simulink model "CrCtl_Governor"  (R2016b)
settings: configuration reference "CodeGenConfigSet" (kept outside this file)
values from neighbouring files (symbols this model uses):
  ACC_ZERO = fi(0,Acc_m_s2)    [init_CrCtl_Governor.m]
  CrCtl_facAcc2TrqCor_C = Calibration.Parameter    [init_CrCtl_Governor.m]
  CrCtl_facDecl2TrqCor_C = Calibration.Parameter    [init_CrCtl_Governor.m]
  CrCtl_facPT11_C = Calibration.Parameter    [init_CrCtl_Governor.m]
  CrCtl_facPT12_C = Calibration.Parameter    [init_CrCtl_Governor.m]
  CrCtl_facPT13_C = Calibration.Parameter    [init_CrCtl_Governor.m]
  CrCtl_facRmpSlpHiAcc_C = Calibration.Parameter    [init_CrCtl_Governor.m]
  CrCtl_facRmpSlpHiDecl_C = Calibration.Parameter    [init_CrCtl_Governor.m]
  CrCtl_facSlpConstRmpDwn_C = Calibration.Parameter    [init_CrCtl_Governor.m]
  CrCtl_facSlpConstRmpUp_C = Calibration.Parameter    [init_CrCtl_Governor.m]
  CrCtl_facSlpRmp1Sus_C = Calibration.Parameter    [init_CrCtl_Governor.m]
  CrCtl_facSlpRmp2Sus_C = Calibration.Parameter    [init_CrCtl_Governor.m]
  CrCtl_facTipDwnCor_CUR = Calibration.Parameter    [init_CrCtl_Governor.m]
  CrCtl_facTipDwnCor_CURX = Calibration.Parameter    [init_CrCtl_Governor.m]
  CrCtl_facTipUpCor_CUR = Calibration.Parameter    [init_CrCtl_Governor.m]
  CrCtl_facTipUpCor_CURX = Calibration.Parameter    [init_CrCtl_Governor.m]
  CrCtl_facTrqIncrSlpConstRmp_C = Calibration.Parameter    [init_CrCtl_Governor.m]
  CrCtl_facTrqIncrTimeConstRmp_C = Calibration.Parameter    [init_CrCtl_Governor.m]
  CrCtl_facTrqRedSlpConstRmp_C = Calibration.Parameter    [init_CrCtl_Governor.m]
  CrCtl_facTrqRedTimeConstRmp_C = Calibration.Parameter    [init_CrCtl_Governor.m]
  CrCtl_facTrqStrtAcc_C = Calibration.Parameter    [init_CrCtl_Governor.m]
  CrCtl_KiAcc1IWin_C = Calibration.Parameter    [init_CrCtl_Governor.m]
  CrCtl_KiAcc2IWin_C = Calibration.Parameter    [init_CrCtl_Governor.m]
  CrCtl_KiAcc3IWin_C = Calibration.Parameter    [init_CrCtl_Governor.m]
  CrCtl_KiCruise1IWin_C = Calibration.Parameter    [init_CrCtl_Governor.m]
  CrCtl_KiCruise2IWin_C = Calibration.Parameter    [init_CrCtl_Governor.m]
  CrCtl_KiCruise3IWin_C = Calibration.Parameter    [init_CrCtl_Governor.m]
  CrCtl_KiDecl1IWin_C = Calibration.Parameter    [init_CrCtl_Governor.m]
  CrCtl_KiDecl2IWin_C = Calibration.Parameter    [init_CrCtl_Governor.m]
  CrCtl_KiDecl3IWin_C = Calibration.Parameter    [init_CrCtl_Governor.m]
  CrCtl_KiNegAcc1IWin_C = Calibration.Parameter    [init_CrCtl_Governor.m]
  CrCtl_KiNegAcc2IWin_C = Calibration.Parameter    [init_CrCtl_Governor.m]
  CrCtl_KiNegAcc3IWin_C = Calibration.Parameter    [init_CrCtl_Governor.m]
  CrCtl_KiNegCruise1IWin_C = Calibration.Parameter    [init_CrCtl_Governor.m]
  CrCtl_KiNegCruise2IWin_C = Calibration.Parameter    [init_CrCtl_Governor.m]
  CrCtl_KiNegCruise3IWin_C = Calibration.Parameter    [init_CrCtl_Governor.m]
  CrCtl_KiNegDecl1IWin_C = Calibration.Parameter    [init_CrCtl_Governor.m]
  CrCtl_KiNegDecl2IWin_C = Calibration.Parameter    [init_CrCtl_Governor.m]
  CrCtl_KiNegDecl3IWin_C = Calibration.Parameter    [init_CrCtl_Governor.m]
  CrCtl_KiNegRes1IWin_C = Calibration.Parameter    [init_CrCtl_Governor.m]
  CrCtl_KiNegRes2IWin_C = Calibration.Parameter    [init_CrCtl_Governor.m]
  CrCtl_KiNegRes3IWin_C = Calibration.Parameter    [init_CrCtl_Governor.m]
  CrCtl_KiNegResCruise1IWin_C = Calibration.Parameter    [init_CrCtl_Governor.m]
  CrCtl_KiNegResCruise2IWin_C = Calibration.Parameter    [init_CrCtl_Governor.m]
  CrCtl_KiNegResCruise3IWin_C = Calibration.Parameter    [init_CrCtl_Governor.m]
  CrCtl_KiPosAcc1IWin_C = Calibration.Parameter    [init_CrCtl_Governor.m]
  CrCtl_KiPosAcc2IWin_C = Calibration.Parameter    [init_CrCtl_Governor.m]
  CrCtl_KiPosAcc3IWin_C = Calibration.Parameter    [init_CrCtl_Governor.m]
  CrCtl_KiPosCruise1IWin_C = Calibration.Parameter    [init_CrCtl_Governor.m]
  CrCtl_KiPosCruise2IWin_C = Calibration.Parameter    [init_CrCtl_Governor.m]
  CrCtl_KiPosCruise3IWin_C = Calibration.Parameter    [init_CrCtl_Governor.m]
  CrCtl_KiPosDecl1IWin_C = Calibration.Parameter    [init_CrCtl_Governor.m]
  CrCtl_KiPosDecl2IWin_C = Calibration.Parameter    [init_CrCtl_Governor.m]
  CrCtl_KiPosDecl3IWin_C = Calibration.Parameter    [init_CrCtl_Governor.m]
  CrCtl_KiPosRes1IWin_C = Calibration.Parameter    [init_CrCtl_Governor.m]
  CrCtl_KiPosRes3IWin_C = Calibration.Parameter    [init_CrCtl_Governor.m]
  CrCtl_KiPosResCruise1IWin_C = Calibration.Parameter    [init_CrCtl_Governor.m]
  CrCtl_KiPosResCruise2IWin_C = Calibration.Parameter    [init_CrCtl_Governor.m]
  CrCtl_KiPosResCruise3IWin_C = Calibration.Parameter    [init_CrCtl_Governor.m]
  CrCtl_KiRes1IWin_C = Calibration.Parameter    [init_CrCtl_Governor.m]
  CrCtl_KiRes2IWin_C = Calibration.Parameter    [init_CrCtl_Governor.m]
  CrCtl_KiRes3IWin_C = Calibration.Parameter    [init_CrCtl_Governor.m]
  CrCtl_KiResCruise1IWin_C = Calibration.Parameter    [init_CrCtl_Governor.m]
  CrCtl_KiResCruise2IWin_C = Calibration.Parameter    [init_CrCtl_Governor.m]
  CrCtl_KiResCruise3IWin_C = Calibration.Parameter    [init_CrCtl_Governor.m]
  CrCtl_KpAcc1PWin_C = Calibration.Parameter    [init_CrCtl_Governor.m]
  CrCtl_KpAcc2PWin_C = Calibration.Parameter    [init_CrCtl_Governor.m]
  CrCtl_KpAcc3PWin_C = Calibration.Parameter    [init_CrCtl_Governor.m]
  CrCtl_KpCruise1PWin_C = Calibration.Parameter    [init_CrCtl_Governor.m]
  CrCtl_KpCruise2PWin_C = Calibration.Parameter    [init_CrCtl_Governor.m]
  CrCtl_KpCruise3PWin_C = Calibration.Parameter    [init_CrCtl_Governor.m]
  CrCtl_KpDecl1PWin_C = Calibration.Parameter    [init_CrCtl_Governor.m]
  CrCtl_KpDecl2PWin_C = Calibration.Parameter    [init_CrCtl_Governor.m]
  CrCtl_KpDecl3PWin_C = Calibration.Parameter    [init_CrCtl_Governor.m]
  CrCtl_KpNegAcc1PWin_C = Calibration.Parameter    [init_CrCtl_Governor.m]
  CrCtl_KpNegAcc2PWin_C = Calibration.Parameter    [init_CrCtl_Governor.m]
  CrCtl_KpNegAcc3PWin_C = Calibration.Parameter    [init_CrCtl_Governor.m]
  CrCtl_KpNegCruise1PWin_C = Calibration.Parameter    [init_CrCtl_Governor.m]
  CrCtl_KpNegCruise2PWin_C = Calibration.Parameter    [init_CrCtl_Governor.m]
  CrCtl_KpNegCruise3PWin_C = Calibration.Parameter    [init_CrCtl_Governor.m]
  CrCtl_KpNegDecl1PWin_C = Calibration.Parameter    [init_CrCtl_Governor.m]
  CrCtl_KpNegDecl2PWin_C = Calibration.Parameter    [init_CrCtl_Governor.m]
  CrCtl_KpNegDecl3PWin_C = Calibration.Parameter    [init_CrCtl_Governor.m]
  CrCtl_KpNegRes1PWin_C = Calibration.Parameter    [init_CrCtl_Governor.m]
  CrCtl_KpNegRes2PWin_C = Calibration.Parameter    [init_CrCtl_Governor.m]
  CrCtl_KpNegRes3PWin_C = Calibration.Parameter    [init_CrCtl_Governor.m]
  CrCtl_KpNegResCruise1PWin_C = Calibration.Parameter    [init_CrCtl_Governor.m]
  CrCtl_KpNegResCruise2PWin_C = Calibration.Parameter    [init_CrCtl_Governor.m]
  CrCtl_KpNegResCruise3PWin_C = Calibration.Parameter    [init_CrCtl_Governor.m]
  CrCtl_KpPosAcc1PWin_C = Calibration.Parameter    [init_CrCtl_Governor.m]
  CrCtl_KpPosAcc2PWin_C = Calibration.Parameter    [init_CrCtl_Governor.m]
  CrCtl_KpPosAcc3PWin_C = Calibration.Parameter    [init_CrCtl_Governor.m]
  CrCtl_KpPosCruise1PWin_C = Calibration.Parameter    [init_CrCtl_Governor.m]
  CrCtl_KpPosCruise2PWin_C = Calibration.Parameter    [init_CrCtl_Governor.m]
  CrCtl_KpPosCruise3PWin_C = Calibration.Parameter    [init_CrCtl_Governor.m]
  CrCtl_KpPosDecl1PWin_C = Calibration.Parameter    [init_CrCtl_Governor.m]
  CrCtl_KpPosDecl2PWin_C = Calibration.Parameter    [init_CrCtl_Governor.m]
  CrCtl_KpPosDecl3PWin_C = Calibration.Parameter    [init_CrCtl_Governor.m]
  CrCtl_KpPosRes1PWin_C = Calibration.Parameter    [init_CrCtl_Governor.m]
  CrCtl_KpPosRes2PWin_C = Calibration.Parameter    [init_CrCtl_Governor.m]
  CrCtl_KpPosRes3PWin_C = Calibration.Parameter    [init_CrCtl_Governor.m]
  CrCtl_KpPosResCruise1PWin_C = Calibration.Parameter    [init_CrCtl_Governor.m]
  CrCtl_KpPosResCruise2PWin_C = Calibration.Parameter    [init_CrCtl_Governor.m]
  CrCtl_KpPosResCruise3PWin_C = Calibration.Parameter    [init_CrCtl_Governor.m]
  CrCtl_KpRes1PWin_C = Calibration.Parameter    [init_CrCtl_Governor.m]
  CrCtl_KpRes2PWin_C = Calibration.Parameter    [init_CrCtl_Governor.m]
  CrCtl_KpRes3PWin_C = Calibration.Parameter    [init_CrCtl_Governor.m]
  CrCtl_KpResCruise1PWin_C = Calibration.Parameter    [init_CrCtl_Governor.m]
  CrCtl_KpResCruise2PWin_C = Calibration.Parameter    [init_CrCtl_Governor.m]
  CrCtl_KpResCruise3PWin_C = Calibration.Parameter    [init_CrCtl_Governor.m]
  CrCtl_numParSelThres1_C = Calibration.Parameter    [init_CrCtl_Governor.m]
  CrCtl_numParSelThres2_C = Calibration.Parameter    [init_CrCtl_Governor.m]
  CrCtl_swtBrkMode_C = Calibration.Parameter    [init_CrCtl_Governor.m]
  CrCtl_swtILimWithP_C = Calibration.Parameter    [init_CrCtl_Governor.m]
  CrCtl_swtOvrRdeFrzInteg_C = Calibration.Parameter    [init_CrCtl_Governor.m]
  CrCtl_swtParSelHysBrk_C = Calibration.Parameter    [init_CrCtl_Governor.m]
  CrCtl_swtPT1EngBrk_C = Calibration.Parameter    [init_CrCtl_Governor.m]
  CrCtl_swtSusRmpInit_C = Calibration.Parameter    [init_CrCtl_Governor.m]
  CrCtl_swtSusRmpStp_C = Calibration.Parameter    [init_CrCtl_Governor.m]
  CrCtl_swtTipUpDwnGvnrStrtVal_C = Calibration.Parameter    [init_CrCtl_Governor.m]
  ... (+88 more)
undefined symbols (not defined in the file or in its folder): CrCtl_Governor_DT, CrCtl_stLck_conv, CrCtl_stOpFunc_conv, CrCtl_stShOff_conv, CrCtl_stSub_conv, CrCtl_stSuspRamp_conv, CruiseCtl_State_conv, EBrk_stPreSelMode_conv, WESDem_State_conv
libraries: CXLib x126, simulink x25
(part 1 of 6)
settings Model: SimulationMode=accelerator  Creator=guanxiaoxing  LastModifiedBy=guanxiaoxing
settings ConfigSetRef: SourceLocation=Base Workspace

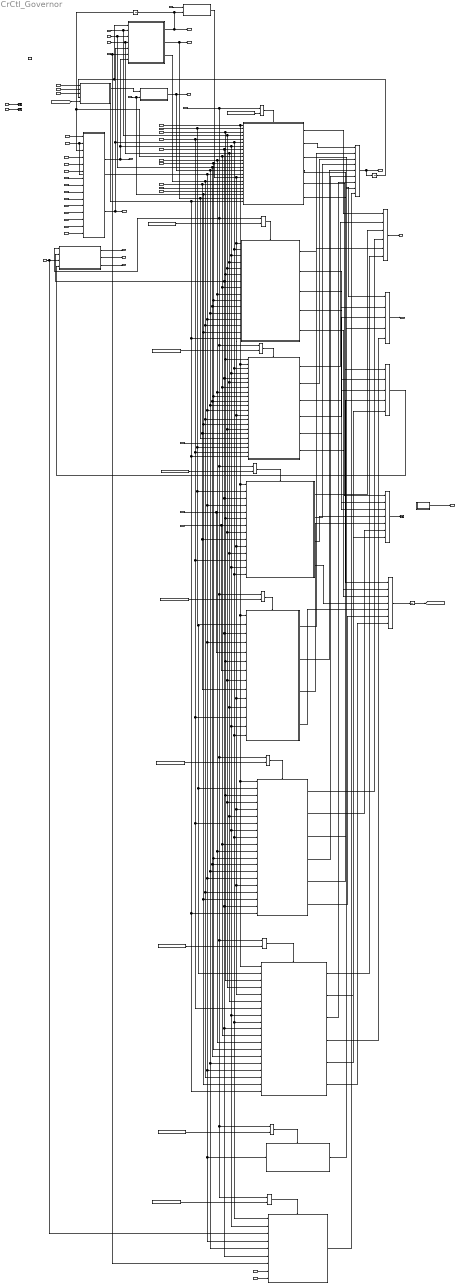
== system CrCtl_Governor ==
  AccPed_trqDes : Inport  Tag=Nm  Description=Driver torque value of propulsion after step limitation  OutMin=-3000  OutMax=3000  OutDataTypeStr=Trq_Nm
  APP_r : Inport  Tag=%  Description=Acceleration pedal sensor 1 value after fault handling  Port=2  OutMin=0  OutMax=100  OutDataTypeStr=Accpedal_rate
  CoETS_trqNTCActvOff : Inport  Tag=Nm  Description=NTC dactivation negative torque  Port=3  OutMin=-3000  OutMax=3000  OutDataTypeStr=Trq_Nm
  CoETS_trqNTCActvOn : Inport  Tag=Nm  Description=NTC activation negative torque  Port=4  OutMin=-3000  OutMax=3000  OutDataTypeStr=Trq_Nm
  CoETS_trqUnFltLtd : Inport  Tag=Nm  Description=Limited idle speed governor torque  Port=5  OutMin=-3276  OutMax=3276  OutDataTypeStr=Trq_Nm
  CoVeh_trqAcs : Inport  Tag=Nm  Description=message for torque demand of accessories  Port=6  OutMin=-3276.8  OutMax=3276.7  OutDataTypeStr=Trq_Nm
  CoVeh_trqPrpLimErr : Inport  Tag=Nm  Description=Limitation torque for propulsion at system error  Port=7  OutMin=-3000  OutMax=3000  OutDataTypeStr=Trq_Nm
  CoVMD_trqLLim : Inport  Tag=Nm  Description=Propulsion torque of longitudinal limiter  Port=8  OutMin=-3000  OutMax=3000  OutDataTypeStr=Trq_Nm
  CrCtl_aAccThres : Inport  Tag=m/s^2  Description=Accelration threshold for Cruise control  Port=9  OutMin=-32  OutMax=32  OutDataTypeStr=Acc_m_s2
  CrCtl_aDeclThres : Inport  Tag=m/s^2  Description=Deaccelration threshold for Cruise control  Port=10  OutMin=-32  OutMax=32  OutDataTypeStr=Acc_m_s2
  CrCtl_st : Inport  Description=Application parameter for Cruise Control state  Port=11  OutDataTypeStr=Enum: CruiseCtl_State_conv
  CrCtl_stGvnr : Inport  Description=Governor status for cruise control  Port=12  OutDataTypeStr=Enum: CruiseCtl_State_conv
  CrCtl_stLck : Inport  Description=Governor status for cruise control  Port=13  OutDataTypeStr=Enum: CrCtl_stLck_conv
  CrCtl_stShOff : Inport  Description=cruise control shut-off requirement  Port=14  OutDataTypeStr=Enum: CrCtl_stShOff_conv
  CrCtl_stSub : Inport  Description=Cruise control sub mode  Port=15  OutDataTypeStr=Enum: CrCtl_stSub_conv
  CrCtl_stSubGvnr : Inport  Description=Cruise control sub mode for governor  Port=16  OutDataTypeStr=Enum: CrCtl_stSub_conv
  CrCtl_stSuspAct : Inport  Description=Cruise Control suspend mode active Status  Port=17  OutMin=0  OutMax=1  OutDataTypeStr=boolean
  CrCtl_stVDirChng : Inport  Description=Flag indicating if vehicle was under increasing speed request before and now speed decrease has been request (or vice-versa).  Port=18  OutMin=0  OutMax=1  OutDataTypeStr=boolean
  CrCtl_vDes : Inport  Tag=km/h  Description=Cruise Control desired set point speed  Port=19  OutMin=0  OutMax=250  OutDataTypeStr=VehSpeed_km_h
  CrCtl_vDesAct : Inport  Tag=km/h  Description=Target speed for cruise control  Port=20  OutMin=0  OutMax=250  OutDataTypeStr=VehSpeed_km_h
  CrCtl_vDesActOld : Inport  Tag=km/h  Description=Cruise control old active speed  Port=21  OutMin=0  OutMax=250  OutDataTypeStr=VehSpeed_km_h
  CrCtl_vMaxDvtAcc : Inport  Tag=km/h  Description=Maximum deviation speed for acceleration  Port=22  OutMin=0  OutMax=250  OutDataTypeStr=VehSpeed_km_h
  CrCtl_vMaxDvtDecl : Inport  Tag=km/h  Description=Maximum deviation speed for deacceleration  Port=23  OutMin=0  OutMax=250  OutDataTypeStr=VehSpeed_km_h
  CrCtl_vMin : Inport  Tag=km/h  Description=Minimum spped for cruise control  Port=24  OutMin=0  OutMax=250  OutDataTypeStr=VehSpeed_km_h
  EBrk_stPreSelMode : Inport  Description=Status of Engine Brake Pre-Selection modes  Port=25  OutDataTypeStr=Enum: EBrk_stPreSelMode_conv
  EngDem_trqInrLim : Inport  Tag=Nm  Description=Resulting limiting torque (inner engine torque)  Port=26  OutMin=-3276.8  OutMax=3276.7  OutDataTypeStr=Trq_Nm
  GlbDa_aXFlt : Inport  Tag=m/s^2  Description=Vehicle longitudinal acceleration filtered  Port=27  OutMin=-32  OutMax=32  OutDataTypeStr=Acc_m_s2
  GlbDa_vXFlt : Inport  Tag=km/h  Description=Vehicle velocity filtered  Port=28  OutMin=0  OutMax=250  OutDataTypeStr=VehSpeed_km_h
  InjSys_trqLim : Inport  Tag=Nm  Description=Torque limitation of injection system  Port=29  OutMin=-3276.8  OutMax=3276.7  OutDataTypeStr=Trq_Nm
  PT_rTraV2N : Inport  Tag=km/h/rpm  Description=Quotient of velocity and engine speed  Port=30  OutMin=-0.32768  OutMax=0.32767  OutDataTypeStr=Tra_V2N_km_h_rpm
  PT_rTrq : Inport  Description=Powertrain torque ratio  Port=31  OutMin=-100  OutMax=100  OutDataTypeStr=TransRatio
  PT_trqLos : Inport  Tag=Nm  Description=Parameter for loss torque of the drive train  Port=32  OutMin=-3000  OutMax=3000  OutDataTypeStr=Trq_Nm
  PT_trqWhl : Inport  Tag=Nm  Description=Actual wheel torque  Port=33  OutMin=-3000  OutMax=3000  OutDataTypeStr=Trq_Nm
  PT_trqWhlMinEng : Inport  Tag=Nm  Description=Minimum wheel torque from the engine  Port=34  OutMin=-3000  OutMax=3000  OutDataTypeStr=Trq_Nm
  PT_trqWhlMinEngBrk : Inport  Tag=Nm  Description=Minimum possible drag torque  Port=35  OutMin=-3000  OutMax=3000  OutDataTypeStr=Trq_Nm
  RngMod_trqMin : Inport  Tag=Nm  Description=Drag torque (minimum torque)  Port=36  OutMin=-3276.8  OutMax=3276.7  OutDataTypeStr=Trq_Nm
  Tra_numGear : Inport  Description=Current gear information  Port=37  OutMin=-128  OutMax=127  OutDataTypeStr=Tra_num
  VehMot_rTrqDfftl : Inport  Description=Torque ratio of differential  Port=38  OutMin=-300  OutMax=300  OutDataTypeStr=TransRatio
  VMD_trqDes : Inport  Tag=Nm  Description=Propulsion torque after driving assistance coordination  Port=39  OutMin=-3000  OutMax=3000  OutDataTypeStr=Trq_Nm
  VMSAdjBtn_st : Inport  Description=Adjustable maximum vehicle Speed limitation button status  Port=40  OutMin=0  OutMax=1  OutDataTypeStr=boolean
  VMSLmtSwt_st : Inport  Description=Vehicle Maximum Speed limit switch value  Port=41  OutMin=0  OutMax=1  OutDataTypeStr=boolean
  WESDem_stCurr : Inport  Description=Status of the working engine Speed Control  Port=42  OutDataTypeStr=Enum: WESDem_State_conv
  function : TriggerPort  TriggerType=function-call  VariantControl=Variant
  Acceleration State : Subsystem
  Constant10 : Constant  Value=CruiseCtl_State_conv.CrCtl_TIP_UP
  Constant11 : Constant  Value=CruiseCtl_State_conv.CrCtl_RESUME_F_BELOW
  Constant12 : Constant  Value=CruiseCtl_State_conv.CrCtl_STAND_BY
  Constant13 : Constant  Value=CruiseCtl_State_conv.CrCtl_OFF
  Constant3 : Constant  Value=CruiseCtl_State_conv.CrCtl_CRUISE
  Constant4 : Constant  Value=CruiseCtl_State_conv.CrCtl_ACCELERATION
  Constant6 : Constant  Value=CruiseCtl_State_conv.CrCtl_DECELERATION
  Constant8 : Constant  Value=CruiseCtl_State_conv.CrCtl_TIP_DOWN
  Constant9 : Constant  Value=CruiseCtl_State_conv.CrCtl_RESUME_F_ABOVE
  CrCtl Engine Brake in v-Hysterisis mode : Subsystem
  Cruise State : Subsystem
  Deceleration State : Subsystem
  Gear Range detection : Subsystem
  Merge : Merge  Inputs=9
  Merge1 : Merge  Inputs=6
  Merge2 : Merge  Inputs=5
  Merge3 : Merge  Inputs=5
  Merge4 : Merge  Inputs=7
  Merge5 : Merge  Inputs=7
  OFF State : Subsystem
  Operating Status Cruise Control : Subsystem
  Relational Operator{,1..8} (9 alike) : RelationalOperator  Operator===  OutDataTypeStr=boolean  RndMeth=Simplest
  Resume From Above : Subsystem
  Resume From Below : Subsystem
  STAND BY State : Subsystem
  Subsystem : Subsystem
  Suspend Request Detection : Subsystem
  Terminator : Terminator
  Terminator1 : Terminator
  Terminator2 : Terminator
  Tip Down State : Subsystem
  Tip Up State : Subsystem
  Unit Delay : UnitDelay  SampleTime=-1
  Unit Delay1 : UnitDelay  SampleTime=-1
  Unit Delay2 : UnitDelay  SampleTime=-1
  Working Range of Cruise Control : Subsystem
  speed limiter status checking : Subsystem
  CrCtl_rTraV2NBeg : Outport  Tag=km/h/rpm  Description=V/N ratio at activation of cruise control  OutMin=-0.32768  OutMax=0.32767  OutDataTypeStr=Tra_V2N_km_h_rpm
  CrCtl_stOpFunc : Outport  Description=state of cruise control operation functionality  Port=2  OutDataTypeStr=Enum: CrCtl_stOpFunc_conv
  CrCtl_stPtd : Outport  Description="Cruise Control is active or on \"\"Stand-BY\"\"-Mode"  Port=3  OutMin=0  OutMax=1  OutDataTypeStr=boolean
  CrCtl_stReq : Outport  Description=Cruise control is active  Port=4  OutMin=0  OutMax=1  OutDataTypeStr=boolean
  CrCtl_stSuspRamp : Outport  Description=Suspend ramp status  Port=5  OutDataTypeStr=Enum: CrCtl_stSuspRamp_conv
  CrCtl_stvHysEngBrkReq : Outport  Description=CrCtl braking status  Port=6  OutMin=0  OutMax=1  OutDataTypeStr=boolean
  CrCtl_trqLead : Outport  Tag=Nm  Description=lead torque of cruise control  Port=7  OutMin=-3000  OutMax=3000  OutDataTypeStr=Trq_Nm
  CrCtl_trqLimAct : Outport  Tag=Nm  Description=Limited Cruise control torque  Port=8  OutMin=-3000  OutMax=3000  OutDataTypeStr=Trq_Nm
  CrCtl_trqMin : Outport  Tag=Nm  Description=cruise control desired torque when cruise control is inactive  Port=9  OutMin=-3000  OutMax=3000  OutDataTypeStr=Trq_Nm
  CrCtl_trqReq : Outport  Tag=Nm  Description=Cruise control torque request  Port=10  OutMin=-3000  OutMax=3000  OutDataTypeStr=Trq_Nm
  CrCtl_trqReqOld : Outport  Tag=Nm  Description=Old Cruise control Governor torque  Port=11  OutMin=-3000  OutMax=3000  OutDataTypeStr=Trq_Nm
  CrCtl_vMax : Outport  Tag=km/h  Description=Maximum speed for cruise control  Port=12  OutMin=0  OutMax=250  OutDataTypeStr=VehSpeed_km_h
  wires:
  Suspend Request Detection/1(CrCtl_trqReqOld) -> CrCtl_trqReqOld/1, Cruise State/12(CrCtl_trqReqOld), Deceleration State/11(CrCtl_trqReqOld), Resume From Above/14(CrCtl_trqReqOld), OFF State/5(CrCtl_trqReqOld), Resume From Below/15(CrCtl_trqReqOld), Acceleration State/14(CrCtl_trqReqOld)  "CrCtl_trqReqOld"
  CrCtl Engine Brake in v-Hysterisis mode/2(CrCtl_vMax) -> Deceleration State/18(CrCtl_vMax), Acceleration State/22(CrCtl_vMax), CrCtl_vMax/1  "CrCtl_vMax"
  CrCtl_aAccThres/1 -> Terminator/1
  CrCtl_aDeclThres/1 -> Terminator1/1
  CrCtl_stShOff/1 -> OFF State/3(CrCtl_stShOff), Operating Status Cruise Control/3(CrCtl_stShOff)
  CrCtl_vDesActOld/1 -> Tip Up State/7(CrCtl_vDesActOld), Tip Down State/7(CrCtl_vDesActOld)
  CrCtl_vMaxDvtDecl/1 -> Deceleration State/19(CrCtl_vMaxDvtDecl)
  Tra_numGear/1 -> Gear Range detection/1(Tra_numGear)
  CoVMD_trqLLim/1 -> speed limiter status checking/3(CoVMD_trqLLim)
  VMSAdjBtn_st/1 -> speed limiter status checking/2(VMSAdjBtn_st)
  VMSLmtSwt_st/1 -> speed limiter status checking/1(VMSLmtSwt_st)
  speed limiter status checking/1(Out1) -> Suspend Request Detection/1(CrCtl_trqReq)
  EBrk_stPreSelMode/1 -> Working Range of Cruise Control/4(EBrk_stPreSelMode)
  PT_trqWhlMinEngBrk/1 -> Working Range of Cruise Control/1(PT_trqWhlMinEngBrk)
  InjSys_trqLim/1 -> Working Range of Cruise Control/5(InjSys_trqLim)
  CoVeh_trqPrpLimErr/1 -> Working Range of Cruise Control/15(CoVeh_trqPrpLimErr)
  CoVeh_trqAcs/1 -> Working Range of Cruise Control/14(CoVeh_trqAcs)
  VehMot_rTrqDfftl/1 -> Working Range of Cruise Control/13(VehMot_rTrqDfftl)
  PT_rTrq/1 -> Working Range of Cruise Control/12(PT_rTrq)
  PT_trqLos/1 -> Working Range of Cruise Control/11(PT_trqLos)
  RngMod_trqMin/1 -> Working Range of Cruise Control/10(RngMod_trqMin)
  CoETS_trqNTCActvOn/1 -> Working Range of Cruise Control/9(CoETS_trqNTCActvOn)
  CoETS_trqNTCActvOff/1 -> Working Range of Cruise Control/8(CoETS_trqNTCActvOff)
  CoETS_trqUnFltLtd/1 -> Working Range of Cruise Control/7(CoETS_trqUnFltLtd)
  EngDem_trqInrLim/1 -> Working Range of Cruise Control/6(EngDem_trqInrLim)
  PT_rTraV2N/1 -> Acceleration State/1(PT_rTraV2N), Resume From Below/1(PT_rTraV2N), Resume From Above/1(PT_rTraV2N), Tip Up State/1(PT_rTraV2N), Tip Down State/1(PT_rTraV2N), Deceleration State/2(PT_rTraV2N)
  WESDem_stCurr/1 -> Resume From Above/2(WESDem_stCurr), Resume From Below/2(WESDem_stCurr), Tip Up State/2(WESDem_stCurr), Tip Down State/2(WESDem_stCurr), Deceleration State/20(WESDem_stCurr), Acceleration State/2(WESDem_stCurr)
  VMD_trqDes/1 -> Cruise State/6(VMD_trqDes), Resume From Below/3(VMD_trqDes), Resume From Above/3(VMD_trqDes), Tip Up State/6(VMD_trqDes), Tip Down State/6(VMD_trqDes), Deceleration State/1(VMD_trqDes), Acceleration State/3(VMD_trqDes)
  PT_trqWhl/1 -> Resume From Below/7(PT_trqWhl), Resume From Above/7(PT_trqWhl), Tip Up State/12(PT_trqWhl), Tip Down State/12(PT_trqWhl), Deceleration State/21(PT_trqWhl), Acceleration State/5(PT_trqWhl)
  APP_r/1 -> Cruise State/9(APP_r), Resume From Below/12(APP_r), Resume From Above/11(APP_r), Deceleration State/8(APP_r), Acceleration State/11(APP_r)
  CrCtl_vMaxDvtAcc/1 -> Acceleration State/20(CrCtl_vMaxDvtAcc)
  GlbDa_aXFlt/1 -> Deceleration State/17(GlbDa_aXFlt), Tip Down State/9(GlbDa_aXFlt), Tip Up State/9(GlbDa_aXFlt), Acceleration State/18(GlbDa_aXFlt)
  AccPed_trqDes/1 -> Cruise State/10(AccPed_trqDes), Resume From Below/13(AccPed_trqDes), Resume From Above/12(AccPed_trqDes), Deceleration State/9(AccPed_trqDes), Acceleration State/12(AccPed_trqDes)
  CrCtl_vMin/1 -> Acceleration State/19(CrCtl_vMin)
  CrCtl Engine Brake in v-Hysterisis mode/1(stvHysEngBrkReq) -> Unit Delay1/1, Gear Range detection/2(stvHysEngBrkReq), CrCtl_stvHysEngBrkReq/1  "CrCtl_stvHysEngBrkReq"
  CrCtl_vDes/1 -> Cruise State/11(CrCtl_vDes), Resume From Below/14(CrCtl_vDes), Resume From Above/13(CrCtl_vDes), Deceleration State/10(CrCtl_vDes), Acceleration State/13(CrCtl_vDes), CrCtl Engine Brake in v-Hysterisis mode/3(CrCtl_vDes)
  CrCtl_st/1 -> OFF State/7(CrCtl_st), CrCtl Engine Brake in v-Hysterisis mode/6(CrCtl_st)
  GlbDa_vXFlt/1 -> Resume From Below/4(GlbDa_vXFlt), Resume From Above/4(GlbDa_vXFlt), Tip Up State/8(GlbDa_vXFlt), Tip Down State/8(GlbDa_vXFlt), Deceleration State/16(GlbDa_vXFlt), Cruise State/5(GlbDa_vXFlt), Acceleration State/4(GlbDa_vXFlt), CrCtl Engine Brake in v-Hysterisis mode/2(GlbDa_vXFlt)
  Operating Status Cruise Control/1(CrCtl_stReq) -> CrCtl_stReq/1  "CrCtl_stReq"
  Operating Status Cruise Control/2(CrCtl_stPtd) -> CrCtl_stPtd/1  "CrCtl_stPtd"
  Operating Status Cruise Control/3(CrCtl_stOpFunc) -> CrCtl_stOpFunc/1  "CrCtl_stOpFunc"
  Working Range of Cruise Control/2(CrCtl_trqLimAct) -> CrCtl_trqLimAct/1, Cruise State/2(CrCtl_trqLimAct), Deceleration State/3(CrCtl_trqLimAct), Tip Down State/14(CrCtl_trqLimAct), OFF State/1(CrCtl_trqLimAct), Resume From Below/9(CrCtl_trqLimAct), Resume From Above/9(CrCtl_trqLimAct), Tip Up State/14(CrCtl_trqLimAct), Acceleration State/6(CrCtl_trqLimAct), CrCtl Engine Brake in v-Hysterisis mode/5(CrCtl_trqLimAct)  "CrCtl_trqLimAct"
  Working Range of Cruise Control/1(CrCtl_trqMin) -> CrCtl Engine Brake in v-Hysterisis mode/7(CrCtl_trqMin), OFF State/2(CrCtl_trqMin), Resume From Below/8(CrCtl_trqMin), Resume From Above/8(CrCtl_trqMin), Tip Up State/13(CrCtl_trqMin), Tip Down State/13(CrCtl_trqMin), Deceleration State/4(CrCtl_trqMin), Cruise State/3(CrCtl_trqMin), Acceleration State/7(CrCtl_trqMin), CrCtl_trqMin/1  "CrCtl_trqMin"
  Merge/1 -> CrCtl_trqReq/1, Unit Delay/1  "CrCtl_trqReq"
  CrCtl_stSuspAct/1 -> Cruise State/15(CrCtl_stSuspAct), Resume From Below/18(CrCtl_stSuspAct), Resume From Above/18(CrCtl_stSuspAct), Deceleration State/15(CrCtl_stSuspAct), Acceleration State/21(CrCtl_stSuspAct), Suspend Request Detection/2(CrCtl_stSuspAct)
  Constant4/1 -> Relational Operator/2
  Relational Operator/1 -> Acceleration State/Enable
  Constant3/1 -> Relational Operator1/2
  Relational Operator1/1 -> Cruise State/Enable
  Constant6/1 -> Relational Operator2/2
  Relational Operator2/1 -> Deceleration State/Enable
  Constant8/1 -> Relational Operator3/2
  Relational Operator3/1 -> Tip Down State/Enable
  Constant9/1 -> Relational Operator4/2
  Relational Operator4/1 -> Resume From Above/Enable
  Constant10/1 -> Relational Operator5/2
  Relational Operator5/1 -> Tip Up State/Enable
  Constant11/1 -> Relational Operator6/2
  Relational Operator6/1 -> Resume From Below/Enable
  Constant12/1 -> Relational Operator7/2
  Relational Operator7/1 -> STAND BY State/Enable
  CrCtl_stGvnr/1 -> Operating Status Cruise Control/1(CrCtl_stGvnr), Relational Operator1/1, Relational Operator8/1, Relational Operator7/1, Relational Operator6/1, Relational Operator4/1, Relational Operator5/1, Relational Operator3/1, Relational Operator2/1, Relational Operator/1
  Constant13/1 -> Relational Operator8/2
  Relational Operator8/1 -> OFF State/Enable
  Gear Range detection/1(CrCtl_stGearRng_mp) -> Deceleration State/13(CrCtl_stGearRng_mp), Resume From Above/5(CrCtl_GearRng_mp), Resume From Below/5(CrCtl_stGearRng_mp), Resume From Above/16(CrCtl_stGearRng_mp), Tip Up State/10(CrCtl_stGearRng_mp), Tip Down State/10(CrCtl_stGearRng_mp), Cruise State/1(CrCtl_stGearRng_mp), Acceleration State/16(CrCtl_stGearRng_mp)
  CrCtl Engine Brake in v-Hysterisis mode/3(stCrCtlOn) -> Cruise State/14(stCrCtlOn), Deceleration State/14(stCrCtlOn), Resume From Below/17(stCrCtlOn), Resume From Above/17(stCrCtlOn), Acceleration State/17(stCrCtlOn)
  CrCtl_stVDirChng/1 -> Tip Up State/5(CrCtl_stVDirChng), Tip Down State/5(CrCtl_stVDirChng)
  CrCtl_vDesAct/1 -> Deceleration State/6(CrCtl_vDesAct), Resume From Below/6(CrCtl_vDesAct), Resume From Above/6(CrCtl_vDesAct), Tip Up State/11(CrCtl_vDesAct), Tip Down State/11(CrCtl_vDesAct), Cruise State/4(CrCtl_vDesAct), Acceleration State/9(CrCtl_vDesAct), CrCtl Engine Brake in v-Hysterisis mode/4(CrCtl_vDesAct)
  PT_trqWhlMinEng/1 -> Deceleration State/12(PT_trqWhlMinEng), Resume From Above/15(PT_trqWhlMinEng), OFF State/4(PT_trqWhlMinEng), STAND BY State/1(PT_trqWhlMinEng), Resume From Below/16(PT_trqWhlMinEng), Tip Up State/4(PT_trqWhlMinEng), Tip Down State/4(PT_trqWhlMinEng), Cruise State/13(PT_trqWhlMinEng), Acceleration State/15(PT_trqWhlMinEng), Working Range of Cruise Control/2(PT_trqWhlMinEng)
  CrCtl_stSubGvnr/1 -> OFF State/6(CrCtl_stSubGvnr), Resume From Below/10(CrCtl_stSubGvnr), Resume From Above/19(CrCtl_stSubGvnr), Tip Up State/3(CrCtl_stSubGvnr), Tip Down State/3(CrCtl_stSubGvnr), Deceleration State/5(CrCtl_stSubGvnr), Cruise State/7(CrCtl_stSubGvnr), Operating Status Cruise Control/2(CrCtl_stSubGvnr), Acceleration State/8(CrCtl_stSubGvnr)
  CrCtl_stSub/1 -> OFF State/8(CrCtl_stSub)
  CrCtl_stLck/1 -> OFF State/9(CrCtl_stLck)
  Unit Delay/1 -> speed limiter status checking/4(CrCtl_trqReq), CrCtl Engine Brake in v-Hysterisis mode/1(CrCtl_trqReq)
  Acceleration State/2(CrCtl_trqReq) -> Merge/1
  Cruise State/1(CrCtl_trqReq) -> Merge/2
  Deceleration State/2(CrCtl_trqReq) -> Merge/3
  Tip Down State/2(CrCtl_trqReq) -> Merge/4
  Tip Up State/2(CrCtl_trqReq) -> Merge/5
  Resume From Above/4(CrCtl_trqReq) -> Merge/6
  Resume From Below/3(CrCtl_trqReq) -> Merge/7
  STAND BY State/1(CrCtl_trqReq) -> Merge/8
  OFF State/1(CrCtl_trqReq) -> Merge/9
  Merge1/1 -> CrCtl_rTraV2NBeg/1  "CrCtl_rTraV2NBeg"
  Acceleration State/1(CrCtl_rTraV2NBeg) -> Merge1/1
  Deceleration State/1(CrCtl_rTraV2NBeg) -> Merge1/2
  Tip Down State/1(CrCtl_rTraV2NBeg) -> Merge1/3
  Resume From Above/1(CrCtl_rTraV2NBeg) -> Merge1/4
  Merge2/1 -> CrCtl_stSuspRamp/1  "CrCtl_stSuspRamp"
  Acceleration State/3(CrCtl_stSuspRamp) -> Merge2/1
  Cruise State/2(CrCtl_stSuspRamp) -> Merge2/2
  Deceleration State/3(CrCtl_stSuspRamp) -> Merge2/3
  Tip Up State/1(CrCtl_rTraV2NBeg) -> Merge1/5
  Resume From Above/3(CrCtl_stSuspRamp) -> Merge2/4
  Resume From Below/1(CrCtl_rTraV2NBeg) -> Merge1/6
  Resume From Below/4(CrCtl_stSuspRamp) -> Merge2/5
  Acceleration State/4(CrCtl_stIWin_mp) -> Merge3/1
  Cruise State/4(CrCtl_stIWin_mp) -> Merge3/2
  Deceleration State/4(CrCtl_stIWin_mp) -> Merge3/3
  Resume From Above/5(CrCtl_stIWin_mp) -> Merge3/4
  Resume From Below/5(CrCtl_stIWin_mp) -> Merge3/5
  Merge3/1 -> Operating Status Cruise Control/4(CrCtl_stIWin_mp)  "CrCtl_stIWin_mp"
  Acceleration State/5(CrCtl_trqReqIWin_mp) -> Merge4/1
  Cruise State/3(CrCtl_trqReqIWin_mp) -> Merge4/2
  Deceleration State/5(CrCtl_trqReqIWin_mp) -> Merge4/3
  Tip Down State/3(CrCtl_trqReqIWin_mp) -> Merge4/4
  Tip Up State/3(CrCtl_trqReqIWin_mp) -> Merge4/5
  Resume From Above/2(CrCtl_trqReqIWin_mp) -> Merge4/6
  Resume From Below/2(CrCtl_trqReqIWin_mp) -> Merge4/7
  Merge4/1 -> Terminator2/1  "CrCtl_trqReqIWin_mp"
  Unit Delay1/1 -> Resume From Below/11(stvHysEngBrkReq), Resume From Above/10(stvHysEngBrkReq), Deceleration State/7(stvHysEngBrkReq), Cruise State/8(stvHysEngBrkReq), Acceleration State/10(stvHysEngBrkReq), Working Range of Cruise Control/3(stvHysEngBrkReq)
  Subsystem/1(Out1) -> CrCtl_trqLead/1  "CrCtl_trqLead"
  Acceleration State/6(CrCtl_trqReqPWin_mp) -> Merge5/1
  Cruise State/5(CrCtl_trqReqPWin_mp) -> Merge5/2
  Deceleration State/6(CrCtl_trqReqPWin_mp) -> Merge5/3
  Tip Down State/4(CrCtl_trqReqPWin_mp) -> Merge5/4
  Tip Up State/4(CrCtl_trqReqPWin_mp) -> Merge5/5
  Resume From Above/6(CrCtl_trqReqPWin_mp) -> Merge5/6
  Resume From Below/6(CrCtl_trqReqPWin_mp) -> Merge5/7
  Merge5/1 -> Unit Delay2/1  "CrCtl_trqReqPWin_mp"
  [CrCtl_trqReqPWin_mp] -> speed limiter status checking/5(CrCtl_trqReqPWin_mp)
  speed limiter status checking/2(Out2) -> Cruise State/16(In1), Deceleration State/22(In1), Resume From Above/20(In1), Resume From Below/19(In1), Acceleration State/23(In1)
  Unit Delay2/1 -> [CrCtl_trqReqPWin_mp]

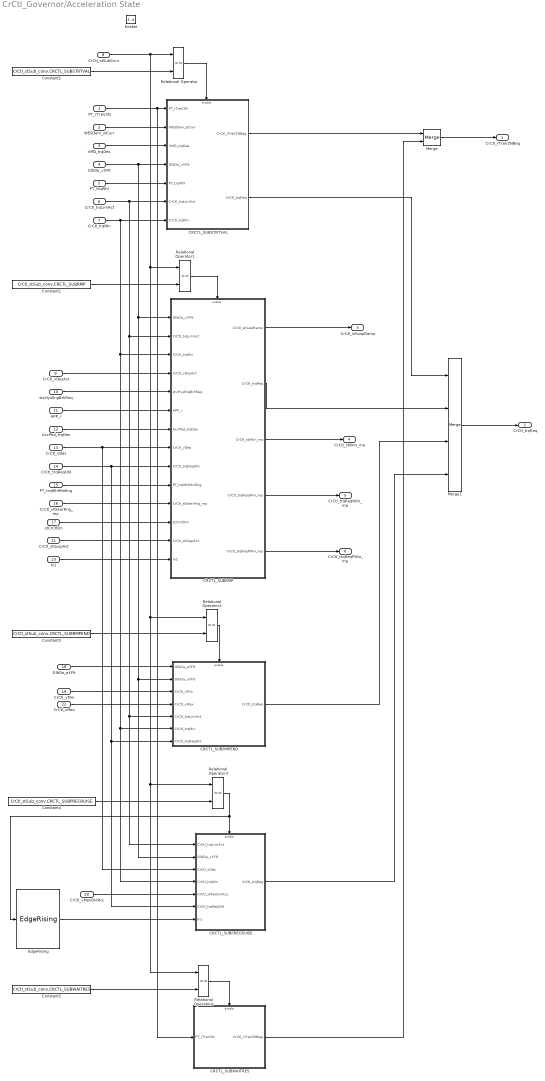
== system CrCtl_Governor/Acceleration State ==
  PT_rTraV2N : Inport
  WESDem_stCurr : Inport  Port=2
  VMD_trqDes : Inport  Port=3
  GlbDa_vXFlt : Inport  Port=4
  PT_trqWhl : Inport  Port=5
  CrCtl_trqLimAct : Inport  Port=6
  CrCtl_trqMin : Inport  Port=7
  CrCtl_stSubGvnr : Inport  Port=8
  CrCtl_vDesAct : Inport  Port=9
  stvHysEngBrkReq : Inport  Port=10
  APP_r : Inport  Port=11
  AccPed_trqDes : Inport  Port=12
  CrCtl_vDes : Inport  Port=13
  CrCtl_trqReqOld : Inport  Port=14
  PT_trqWhlMinEng : Inport  Port=15
  CrCtl_stGearRng_mp : Inport  Port=16
  stCrCtlOn : Inport  Port=17
  GlbDa_aXFlt : Inport  Port=18
  CrCtl_vMin : Inport  Port=19
  CrCtl_vMaxDvtAcc : Inport  Port=20
  CrCtl_stSuspAct : Inport  Port=21
  CrCtl_vMax : Inport  Port=22
  In1 : Inport  Port=23
  Enable : EnablePort
  CRCTL_SUBPRECRUISE : Subsystem
  CRCTL_SUBRMP : Subsystem
  CRCTL_SUBRMPEND : Subsystem
  CRCTL_SUBSTRTVAL : Subsystem
  CRCTL_SUBWAITRES : Subsystem
  Constant1 : Constant  Value=CrCtl_stSub_conv.CRCTL_SUBRMP
  Constant2 : Constant  Value=CrCtl_stSub_conv.CRCTL_SUBSTRTVAL
  Constant3 : Constant  Value=CrCtl_stSub_conv.CRCTL_SUBRMPEND
  Constant4 : Constant  Value=CrCtl_stSub_conv.CRCTL_SUBPRECRUISE
  Constant5 : Constant  Value=CrCtl_stSub_conv.CRCTL_SUBWAITRES
  EdgeRising : CXLib/EdgeRising
  Merge : Merge
  Merge1 : Merge  Inputs=4
  Relational Operator{,1..4} (5 alike) : RelationalOperator  Operator===  OutDataTypeStr=boolean  RndMeth=Simplest
  CrCtl_rTraV2NBeg : Outport
  CrCtl_trqReq : Outport  Port=2
  CrCtl_stSuspRamp : Outport  Port=3
  CrCtl_stIWin_mp : Outport  Port=4
  CrCtl_trqReqIWin_mp : Outport  Port=5
  CrCtl_trqReqPWin_mp : Outport  Port=6
  wires:
  WESDem_stCurr/1 -> CRCTL_SUBSTRTVAL/2(WESDem_stCurr)
  VMD_trqDes/1 -> CRCTL_SUBSTRTVAL/3(VMD_trqDes)
  PT_trqWhl/1 -> CRCTL_SUBSTRTVAL/5(PT_trqWhl)
  CrCtl_vDesAct/1 -> CRCTL_SUBRMP/4(CrCtl_vDesAct)
  stvHysEngBrkReq/1 -> CRCTL_SUBRMP/5(stvHysEngBrkReq)
  APP_r/1 -> CRCTL_SUBRMP/6(APP_r)
  AccPed_trqDes/1 -> CRCTL_SUBRMP/7(AccPed_trqDes)
  stCrCtlOn/1 -> CRCTL_SUBRMP/12(stCrCtlOn)
  CrCtl_stGearRng_mp/1 -> CRCTL_SUBRMP/11(CrCtl_stGearRng_mp)
  PT_trqWhlMinEng/1 -> CRCTL_SUBRMP/10(PT_trqWhlMinEng)
  GlbDa_aXFlt/1 -> CRCTL_SUBRMPEND/1(GlbDa_aXFlt)
  CrCtl_vMin/1 -> CRCTL_SUBRMPEND/3(CrCtl_vMin)
  CrCtl_trqLimAct/1 -> CRCTL_SUBPRECRUISE/1(CrCtl_trqLimAct), CRCTL_SUBRMPEND/5(CrCtl_trqLimAct), CRCTL_SUBRMP/2(CrCtl_trqLimAct), CRCTL_SUBSTRTVAL/6(CrCtl_trqLimAct)
  GlbDa_vXFlt/1 -> CRCTL_SUBPRECRUISE/2(GlbDa_vXFlt), CRCTL_SUBRMPEND/2(GlbDa_vXFlt), CRCTL_SUBRMP/1(GlbDa_vXFlt), CRCTL_SUBSTRTVAL/4(GlbDa_vXFlt)
  CrCtl_vDes/1 -> CRCTL_SUBPRECRUISE/3(CrCtl_vDes), CRCTL_SUBRMP/8(CrCtl_vDes)
  CrCtl_trqMin/1 -> CRCTL_SUBPRECRUISE/4(CrCtl_trqMin), CRCTL_SUBRMPEND/6(CrCtl_trqMin), CRCTL_SUBRMP/3(CrCtl_trqMin), CRCTL_SUBSTRTVAL/7(CrCtl_trqMin)
  CrCtl_vMaxDvtAcc/1 -> CRCTL_SUBPRECRUISE/5(CrCtl_vMaxDvtAcc)
  PT_rTraV2N/1 -> CRCTL_SUBWAITRES/1(PT_rTraV2N), CRCTL_SUBSTRTVAL/1(PT_rTraV2N)
  CrCtl_stSuspAct/1 -> CRCTL_SUBRMP/13(CrCtl_stSuspAct)
  Constant2/1 -> Relational Operator/2
  Relational Operator/1 -> CRCTL_SUBSTRTVAL/Enable
  Constant1/1 -> Relational Operator1/2
  Relational Operator1/1 -> CRCTL_SUBRMP/Enable
  Constant3/1 -> Relational Operator2/2
  Relational Operator2/1 -> CRCTL_SUBRMPEND/Enable
  Constant4/1 -> Relational Operator3/2
  Relational Operator3/1 -> EdgeRising/1, CRCTL_SUBPRECRUISE/Enable
  CrCtl_stSubGvnr/1 -> Relational Operator4/1, Relational Operator3/1, Relational Operator2/1, Relational Operator1/1, Relational Operator/1
  Constant5/1 -> Relational Operator4/2
  Relational Operator4/1 -> CRCTL_SUBWAITRES/Enable
  CrCtl_vMax/1 -> CRCTL_SUBRMPEND/4(CrCtl_vMax)
  CrCtl_trqReqOld/1 -> CRCTL_SUBPRECRUISE/6(CrCtl_trqReqOld), CRCTL_SUBRMPEND/7(CrCtl_trqReqOld), CRCTL_SUBRMP/9(CrCtl_trqReqOld)
  CRCTL_SUBSTRTVAL/1(CrCtl_rTraV2NBeg) -> Merge/1
  Merge/1 -> CrCtl_rTraV2NBeg/1
  CRCTL_SUBRMP/3(CrCtl_stIWin_mp) -> CrCtl_stIWin_mp/1
  CRCTL_SUBRMP/4(CrCtl_trqReqIWin_mp) -> CrCtl_trqReqIWin_mp/1
  CRCTL_SUBRMP/1(CrCtl_stSuspRamp) -> CrCtl_stSuspRamp/1
  Merge1/1 -> CrCtl_trqReq/1
  CRCTL_SUBRMP/2(CrCtl_trqReq) -> Merge1/2
  CRCTL_SUBSTRTVAL/2(CrCtl_trqReq) -> Merge1/1
  CRCTL_SUBRMPEND/1(CrCtl_trqReq) -> Merge1/3
  CRCTL_SUBPRECRUISE/1(CrCtl_trqReq) -> Merge1/4
  CRCTL_SUBWAITRES/1(CrCtl_rTraV2NBeg) -> Merge/2
  EdgeRising/1 -> CRCTL_SUBPRECRUISE/7(In1)
  CRCTL_SUBRMP/5(CrCtl_trqReqPWin_mp) -> CrCtl_trqReqPWin_mp/1
  In1/1 -> CRCTL_SUBRMP/14(In2)

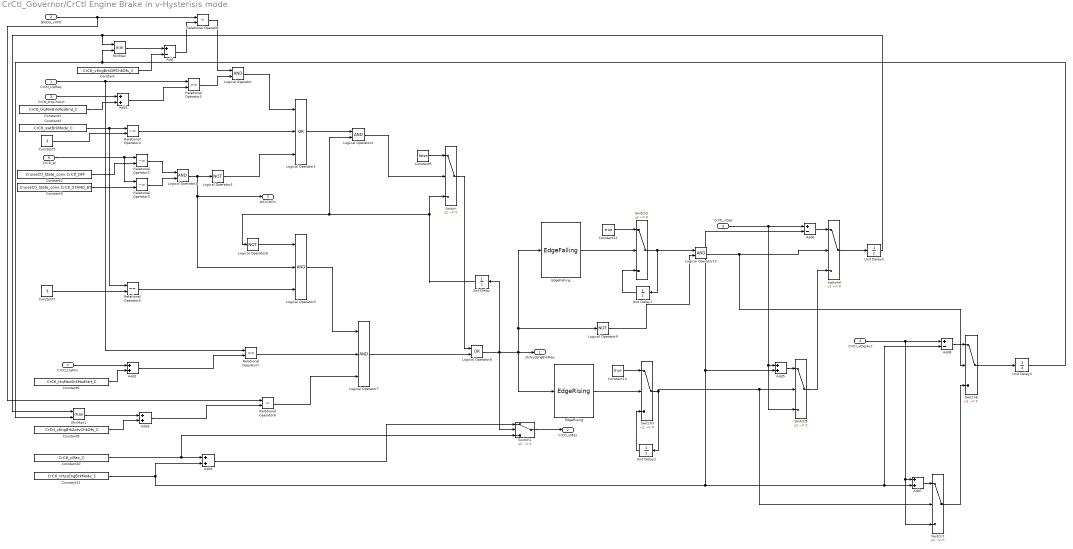
== system CrCtl_Governor/CrCtl Engine Brake in v-Hysterisis mode ==
  CrCtl_trqReq : Inport
  GlbDa_vXFlt : Inport  Port=2
  CrCtl_vDes : Inport  Port=3
  CrCtl_vDesAct : Inport  Port=4
  CrCtl_trqLimAct : Inport  Port=5
  CrCtl_st : Inport  Port=6
  CrCtl_trqMin : Inport  Port=7
  Add : Sum  Inputs=+-
  Add{1..5,7} (6 alike) : Sum
  Add6 : Sum  Inputs=+-
  Add8 : Sum  Inputs=+-
  Constant : Constant  Value=CrCtl_vEngBrkOffChkOfs_C
  Constant1 : Constant  Value=CrCtl_trqMinBrkModEnd_C
  Constant10 : Constant  Value=CrCtl_vMax_C
  Constant11 : Constant  Value=CrCtl_vHysEngBrkMode_C
  Constant12 : Constant  Value=true
  Constant13 : Constant  Value=true
  Constant2 : Constant  Value=CruiseCtl_State_conv.CrCtl_OFF
  Constant3 : Constant  Value=CruiseCtl_State_conv.CrCtl_STAND_BY
  Constant4 : Constant  Value=CrCtl_swtBrkMode_C
  Constant5 : Constant  Value=3  OutDataTypeStr=State_uint8
  Constant6 : Constant  Value=CrCtl_trqMaxBrkModStrt_C
  Constant7 : Constant  Value=3  OutDataTypeStr=State_uint8
  Constant8 : Constant  Value=CrCtl_vEngBrkActvChkOfs_C
  Constant9 : Constant  Value=false
  EdgeFalling : CXLib/EdgeFalling
  EdgeRising : CXLib/EdgeRising
  Logical Operator{,2,4,10} (4 alike) : Logic  AllPortsSameDT=off  OutDataTypeStr=boolean
  Logical Operator1 : Logic  Operator=OR  Inputs=3  AllPortsSameDT=off  OutDataTypeStr=boolean
  Logical Operator3 : Logic  Operator=NOT  AllPortsSameDT=off  OutDataTypeStr=boolean
  Logical Operator5 : Logic  Inputs=3  AllPortsSameDT=off  OutDataTypeStr=boolean
  Logical Operator6 : Logic  Operator=NOT  AllPortsSameDT=off  OutDataTypeStr=boolean
  Logical Operator7 : Logic  Inputs=3  AllPortsSameDT=off  OutDataTypeStr=boolean
  Logical Operator8 : Logic  Operator=OR  AllPortsSameDT=off  OutDataTypeStr=boolean
  Logical Operator9 : Logic  Operator=NOT  AllPortsSameDT=off  OutDataTypeStr=boolean
  MinMax : MinMax  Inputs=2
  MinMax1 : MinMax  Function=max  Inputs=2
  Relational Operator : RelationalOperator  Operator=<  OutDataTypeStr=boolean  RndMeth=Simplest
  Relational Operator1 : RelationalOperator  OutDataTypeStr=boolean  RndMeth=Simplest
  Relational Operator2 : RelationalOperator  Operator=~=  OutDataTypeStr=boolean  RndMeth=Simplest
  Relational Operator3 : RelationalOperator  Operator=~=  OutDataTypeStr=boolean  RndMeth=Simplest
  Relational Operator4 : RelationalOperator  Operator=~=  OutDataTypeStr=boolean  RndMeth=Simplest
  Relational Operator5 : RelationalOperator  Operator===  OutDataTypeStr=boolean  RndMeth=Simplest
  Relational Operator6 : RelationalOperator  Operator=>  OutDataTypeStr=boolean  RndMeth=Simplest
  Relational Operator7 : RelationalOperator  Operator=<=  OutDataTypeStr=boolean  RndMeth=Simplest
  Switch{,1..7} (8 alike) : Switch  Criteria=u2 ~= 0
  Unit Delay{,1..4} (5 alike) : UnitDelay  SampleTime=-1
  stvHysEngBrkReq : Outport
  CrCtl_vMax : Outport  Port=2
  stCrCtlOn : Outport  Port=3
  wires:
  GlbDa_vXFlt/1 -> Relational Operator6/1, Relational Operator/1
  MinMax/1 -> Add/1
  Constant/1 -> Add/2
  Add/1 -> Relational Operator/2
  Relational Operator/1 -> Logical Operator/1
  CrCtl_trqLimAct/1 -> Add1/1
  Constant1/1 -> Add1/2
  Add1/1 -> Relational Operator1/2
  Relational Operator1/1 -> Logical Operator/2
  Logical Operator/1 -> Logical Operator1/1
  CrCtl_st/1 -> Relational Operator3/1, Relational Operator2/1
  Constant2/1 -> Relational Operator2/2
  Constant3/1 -> Relational Operator3/2
  Relational Operator2/1 -> Logical Operator2/1
  Relational Operator3/1 -> Logical Operator2/2
  Constant5/1 -> Relational Operator4/2
  Relational Operator4/1 -> Logical Operator1/2
  Logical Operator3/1 -> Logical Operator1/3
  Logical Operator1/1 -> Logical Operator4/1
  Constant4/1 -> Relational Operator5/1, Relational Operator4/1
  Constant7/1 -> Relational Operator5/2
  Relational Operator5/1 -> Logical Operator5/3
  Logical Operator6/1 -> Logical Operator5/1
  Logical Operator5/1 -> Logical Operator7/1
  Relational Operator7/1 -> Logical Operator7/2
  CrCtl_trqReq/1 -> Relational Operator7/1, Relational Operator1/1
  Add2/1 -> Relational Operator7/2
  Constant6/1 -> Add2/2
  CrCtl_trqMin/1 -> Add2/1
  Relational Operator6/1 -> Logical Operator7/3
  MinMax1/1 -> Add3/1
  Constant8/1 -> Add3/2
  Add3/1 -> Relational Operator6/2
  Switch4/1 -> Unit Delay3/1
  Switch6/1 -> Unit Delay4/1
  Logical Operator7/1 -> Logical Operator8/2
  Logical Operator4/1 -> Switch/2
  Constant9/1 -> Switch/1
  Switch/1 -> Logical Operator8/1
  Constant10/1 -> Switch1/3, Add4/1
  Logical Operator8/1 -> Switch1/2, EdgeRising/1, Logical Operator9/1, EdgeFalling/1, stvHysEngBrkReq/1, Unit Delay/1
  Add4/1 -> Switch1/1
  Switch1/1 -> CrCtl_vMax/1
  Logical Operator2/1 -> stCrCtlOn/1, Logical Operator5/2, Logical Operator3/1
  Unit Delay/1 -> Logical Operator4/2, Logical Operator6/1, Switch/3
  EdgeRising/1 -> Switch3/2
  EdgeFalling/1 -> Switch2/2
  Constant12/1 -> Switch2/1
  Unit Delay1/1 -> Switch2/3
  Add6/1 -> Switch4/1
  CrCtl_vDes/1 -> Switch5/3, Add5/1, Add6/1
  Unit Delay2/1 -> Switch3/3
  Constant13/1 -> Switch3/1
  Add5/1 -> Switch5/1
  Switch5/1 -> Switch4/3
  Switch2/1 -> Logical Operator10/1, Unit Delay1/1
  Constant11/1 -> Add7/2, Add8/2, Add5/2, Add6/2, Add4/2
  Add8/1 -> Switch6/1
  CrCtl_vDesAct/1 -> Switch7/3, Add7/1, Add8/1
  Switch3/1 -> Switch7/2, Switch5/2, Unit Delay2/1
  Add7/1 -> Switch7/1
  Switch7/1 -> Switch6/3
  Logical Operator9/1 -> Logical Operator10/2
  Logical Operator10/1 -> Switch6/2, Switch4/2
  Unit Delay3/1 -> MinMax1/1, MinMax/1
  Unit Delay4/1 -> MinMax1/2, MinMax/2

== system CrCtl_Governor/Cruise State ==
  CrCtl_stGearRng_mp : Inport
  CrCtl_trqLimAct : Inport  Port=2
  CrCtl_trqMin : Inport  Port=3
  CrCtl_vDesAct : Inport  Port=4
  GlbDa_vXFlt : Inport  Port=5
  VMD_trqDes : Inport  Port=6
  CrCtl_stSubGvnr : Inport  Port=7
  stvHysEngBrkReq : Inport  Port=8
  APP_r : Inport  Port=9
  AccPed_trqDes : Inport  Port=10
  CrCtl_vDes : Inport  Port=11
  CrCtl_trqReqOld : Inport  Port=12
  PT_trqWhlMinEng : Inport  Port=13
  stCrCtlOn : Inport  Port=14
  CrCtl_stSuspAct : Inport  Port=15
  In1 : Inport  Port=16
  Enable : EnablePort
  CRCTL_SUBGVNR : Subsystem
  CRCTL_SUBSTRTVAL : Subsystem
  Constant1 : Constant  Value=CrCtl_stSub_conv.CRCTL_SUBSTRTVAL
  Constant2 : Constant  Value=CrCtl_stSub_conv.CRCTL_SUBGVNR
  Merge : Merge
  Relational Operator1 : RelationalOperator  Operator===  OutDataTypeStr=boolean  RndMeth=Simplest
  Relational Operator2 : RelationalOperator  Operator===  OutDataTypeStr=boolean  RndMeth=Simplest
  CrCtl_trqReq : Outport
  CrCtl_stSuspRamp : Outport  Port=2
  CrCtl_trqReqIWin_mp : Outport  Port=3
  CrCtl_stIWin_mp : Outport  Port=4
  CrCtl_trqReqPWin_mp : Outport  Port=5
  wires:
  Constant1/1 -> Relational Operator1/2
  Relational Operator1/1 -> CRCTL_SUBSTRTVAL/Enable
  CrCtl_stSubGvnr/1 -> Relational Operator2/1, Relational Operator1/1
  Constant2/1 -> Relational Operator2/2
  Relational Operator2/1 -> CRCTL_SUBGVNR/Enable
  CrCtl_trqLimAct/1 -> CRCTL_SUBGVNR/2(CrCtl_trqLimAct), CRCTL_SUBSTRTVAL/2(CrCtl_trqLimAct)
  CrCtl_trqMin/1 -> CRCTL_SUBGVNR/3(CrCtl_trqMin), CRCTL_SUBSTRTVAL/3(CrCtl_trqMin)
  CrCtl_vDesAct/1 -> CRCTL_SUBGVNR/4(CrCtl_vDesAct), CRCTL_SUBSTRTVAL/4(CrCtl_vDesAct)
  GlbDa_vXFlt/1 -> CRCTL_SUBGVNR/1(GlbDa_vXFlt), CRCTL_SUBSTRTVAL/5(GlbDa_vXFlt)
  VMD_trqDes/1 -> CRCTL_SUBSTRTVAL/6(VMD_trqDes)
  stvHysEngBrkReq/1 -> CRCTL_SUBGVNR/5(stvHysEngBrkReq)
  APP_r/1 -> CRCTL_SUBGVNR/6(APP_r)
  AccPed_trqDes/1 -> CRCTL_SUBGVNR/7(AccPed_trqDes)
  stCrCtlOn/1 -> CRCTL_SUBGVNR/12(stCrCtlOn)
  CrCtl_stGearRng_mp/1 -> CRCTL_SUBGVNR/11(CrCtl_stGearRng_mp), CRCTL_SUBSTRTVAL/1(CrCtl_stGearRng_mp)
  PT_trqWhlMinEng/1 -> CRCTL_SUBGVNR/10(PT_trqWhlMinEng)
  CrCtl_vDes/1 -> CRCTL_SUBGVNR/8(CrCtl_vDes)
  CrCtl_stSuspAct/1 -> CRCTL_SUBGVNR/13(CrCtl_stSuspAct)
  CrCtl_trqReqOld/1 -> CRCTL_SUBGVNR/9(CrCtl_trqReqOld)
  Merge/1 -> CrCtl_trqReq/1
  CRCTL_SUBSTRTVAL/1(CrCtl_trqReq) -> Merge/1
  CRCTL_SUBGVNR/2(CrCtl_trqReq) -> Merge/2
  CRCTL_SUBGVNR/1(CrCtl_stSuspRamp) -> CrCtl_stSuspRamp/1
  CRCTL_SUBGVNR/4(CrCtl_trqReqIWin_mp) -> CrCtl_trqReqIWin_mp/1
  CRCTL_SUBGVNR/3(CrCtl_stIWin_mp) -> CrCtl_stIWin_mp/1
  CRCTL_SUBGVNR/5(CrCtl_trqReqPWin_mp) -> CrCtl_trqReqPWin_mp/1
  In1/1 -> CRCTL_SUBGVNR/14(In2)

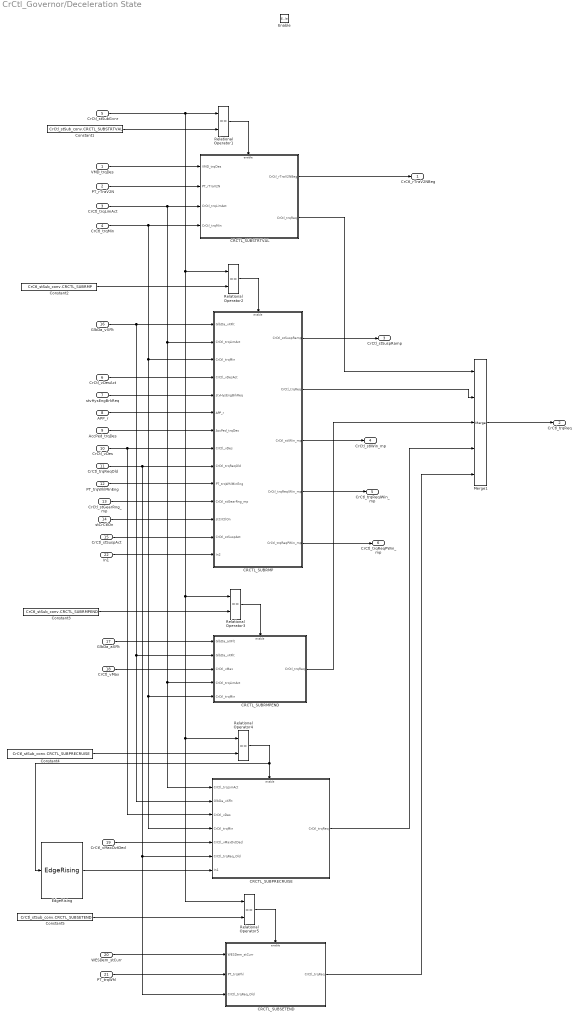
== system CrCtl_Governor/Deceleration State ==
  VMD_trqDes : Inport
  PT_rTraV2N : Inport  Port=2
  CrCtl_trqLimAct : Inport  Port=3
  CrCtl_trqMin : Inport  Port=4
  CrCtl_stSubGvnr : Inport  Port=5
  CrCtl_vDesAct : Inport  Port=6
  stvHysEngBrkReq : Inport  Port=7
  APP_r : Inport  Port=8
  AccPed_trqDes : Inport  Port=9
  CrCtl_vDes : Inport  Port=10
  CrCtl_trqReqOld : Inport  Port=11
  PT_trqWhlMinEng : Inport  Port=12
  CrCtl_stGearRng_mp : Inport  Port=13
  stCrCtlOn : Inport  Port=14
  CrCtl_stSuspAct : Inport  Port=15
  GlbDa_vXFlt : Inport  Port=16
  GlbDa_aXFlt : Inport  Port=17
  CrCtl_vMax : Inport  Port=18
  CrCtl_vMaxDvtDecl : Inport  Port=19
  WESDem_stCurr : Inport  Port=20
  PT_trqWhl : Inport  Port=21
  In1 : Inport  Port=22
  Enable : EnablePort
  CRCTL_SUBPRECRUISE : Subsystem
  CRCTL_SUBRMP : Subsystem
  CRCTL_SUBRMPEND : Subsystem
  CRCTL_SUBSETEND : Subsystem
  CRCTL_SUBSTRTVAL : Subsystem
  Constant1 : Constant  Value=CrCtl_stSub_conv.CRCTL_SUBSTRTVAL
  Constant2 : Constant  Value=CrCtl_stSub_conv.CRCTL_SUBRMP
  Constant3 : Constant  Value=CrCtl_stSub_conv.CRCTL_SUBRMPEND
  Constant4 : Constant  Value=CrCtl_stSub_conv.CRCTL_SUBPRECRUISE
  Constant5 : Constant  Value=CrCtl_stSub_conv.CRCTL_SUBSETEND
  EdgeRising : CXLib/EdgeRising
  Merge1 : Merge  Inputs=5
  Relational Operator{1..5} (5 alike) : RelationalOperator  Operator===  OutDataTypeStr=boolean  RndMeth=Simplest
  CrCtl_rTraV2NBeg : Outport
  CrCtl_trqReq : Outport  Port=2
  CrCtl_stSuspRamp : Outport  Port=3
  CrCtl_stIWin_mp : Outport  Port=4
  CrCtl_trqReqIWin_mp : Outport  Port=5
  CrCtl_trqReqPWin_mp : Outport  Port=6
  wires:
  PT_rTraV2N/1 -> CRCTL_SUBSTRTVAL/2(PT_rTraV2N)
  VMD_trqDes/1 -> CRCTL_SUBSTRTVAL/1(VMD_trqDes)
  Constant1/1 -> Relational Operator1/2
  Relational Operator1/1 -> CRCTL_SUBSTRTVAL/Enable
  Constant2/1 -> Relational Operator2/2
  Relational Operator2/1 -> CRCTL_SUBRMP/Enable
  Constant3/1 -> Relational Operator3/2
  Relational Operator3/1 -> CRCTL_SUBRMPEND/Enable
  Constant4/1 -> Relational Operator4/2
  Relational Operator4/1 -> EdgeRising/1, CRCTL_SUBPRECRUISE/Enable
  CrCtl_stSubGvnr/1 -> Relational Operator1/1, Relational Operator3/1, Relational Operator4/1, Relational Operator5/1, Relational Operator2/1
  Constant5/1 -> Relational Operator5/2
  Relational Operator5/1 -> CRCTL_SUBSETEND/Enable
  CrCtl_vDesAct/1 -> CRCTL_SUBRMP/4(CrCtl_vDesAct)
  stvHysEngBrkReq/1 -> CRCTL_SUBRMP/5(stvHysEngBrkReq)
  APP_r/1 -> CRCTL_SUBRMP/6(APP_r)
  AccPed_trqDes/1 -> CRCTL_SUBRMP/7(AccPed_trqDes)
  stCrCtlOn/1 -> CRCTL_SUBRMP/12(stCrCtlOn)
  CrCtl_stGearRng_mp/1 -> CRCTL_SUBRMP/11(CrCtl_stGearRng_mp)
  PT_trqWhlMinEng/1 -> CRCTL_SUBRMP/10(PT_trqWhlMinEng)
  CrCtl_stSuspAct/1 -> CRCTL_SUBRMP/13(CrCtl_stSuspAct)
  GlbDa_vXFlt/1 -> CRCTL_SUBRMP/1(GlbDa_vXFlt), CRCTL_SUBPRECRUISE/2(GlbDa_vXFlt), CRCTL_SUBRMPEND/2(GlbDa_vXFlt)
  GlbDa_aXFlt/1 -> CRCTL_SUBRMPEND/1(GlbDa_aXFlt)
  CrCtl_vMax/1 -> CRCTL_SUBRMPEND/3(CrCtl_vMax)
  CrCtl_trqMin/1 -> CRCTL_SUBSTRTVAL/4(CrCtl_trqMin), CRCTL_SUBPRECRUISE/4(CrCtl_trqMin), CRCTL_SUBRMPEND/5(CrCtl_trqMin), CRCTL_SUBRMP/3(CrCtl_trqMin)
  CrCtl_trqLimAct/1 -> CRCTL_SUBRMPEND/4(CrCtl_trqLimAct), CRCTL_SUBPRECRUISE/1(CrCtl_trqLimAct), CRCTL_SUBRMP/2(CrCtl_trqLimAct), CRCTL_SUBSTRTVAL/3(CrCtl_trqLimAct)
  CrCtl_vDes/1 -> CRCTL_SUBPRECRUISE/3(CrCtl_vDes), CRCTL_SUBRMP/8(CrCtl_vDes)
  CrCtl_vMaxDvtDecl/1 -> CRCTL_SUBPRECRUISE/5(CrCtl_vMaxDvtDecl)
  CrCtl_trqReqOld/1 -> CRCTL_SUBSETEND/3(CrCtl_trqReq_Old), CRCTL_SUBPRECRUISE/6(CrCtl_trqReq_Old), CRCTL_SUBRMP/9(CrCtl_trqReqOld)
  WESDem_stCurr/1 -> CRCTL_SUBSETEND/1(WESDem_stCurr)
  PT_trqWhl/1 -> CRCTL_SUBSETEND/2(PT_trqWhl)
  CRCTL_SUBSTRTVAL/1(CrCtl_rTraV2NBeg) -> CrCtl_rTraV2NBeg/1
  CRCTL_SUBRMP/3(CrCtl_stIWin_mp) -> CrCtl_stIWin_mp/1
  CRCTL_SUBRMP/4(CrCtl_trqReqIWin_mp) -> CrCtl_trqReqIWin_mp/1
  CRCTL_SUBRMP/1(CrCtl_stSuspRamp) -> CrCtl_stSuspRamp/1
  Merge1/1 -> CrCtl_trqReq/1
  CRCTL_SUBRMP/2(CrCtl_trqReq) -> Merge1/2
  CRCTL_SUBSTRTVAL/2(CrCtl_trqReq) -> Merge1/1
  CRCTL_SUBRMPEND/1(CrCtl_trqReq) -> Merge1/3
  CRCTL_SUBPRECRUISE/1(CrCtl_trqReq) -> Merge1/4
  CRCTL_SUBSETEND/1(CrCtl_trqReq) -> Merge1/5
  EdgeRising/1 -> CRCTL_SUBPRECRUISE/7(In1)
  CRCTL_SUBRMP/5(CrCtl_trqReqPWin_mp) -> CrCtl_trqReqPWin_mp/1
  In1/1 -> CRCTL_SUBRMP/14(In2)

== system CrCtl_Governor/Gear Range detection ==
  Tra_numGear : Inport
  stvHysEngBrkReq : Inport  Port=2
  Constant : Constant  Value=CrCtl_numParSelThres1_C
  Constant1 : Constant  Value=CrCtl_numParSelThres2_C
  Constant2 : Constant  Value=PIGVNRSET2
  Constant3 : Constant  Value=PIGVNRSET3
  Constant4 : Constant  Value=PIGVNRSET1
  Constant5 : Constant  Value=CrCtl_swtParSelHysBrk_C
  Multiport Switch : MultiPortSwitch  DataPortOrder=Zero-based contiguous  Inputs=4
  Relational Operator : RelationalOperator  Operator=<  OutDataTypeStr=boolean  RndMeth=Simplest
  Relational Operator1 : RelationalOperator  Operator=>  OutDataTypeStr=boolean  RndMeth=Simplest
  Switch : Switch  Criteria=u2 ~= 0
  Switch1 : Switch  Criteria=u2 ~= 0
  Switch2 : Switch  Criteria=u2 ~= 0
  CrCtl_stGearRng_mp : Outport
  wires:
  Constant/1 -> Relational Operator/2
  Tra_numGear/1 -> Relational Operator1/1, Relational Operator/1
  Constant1/1 -> Relational Operator1/2
  Relational Operator1/1 -> Switch/2
  Relational Operator/1 -> Switch1/2
  Constant4/1 -> Multiport Switch/3, Switch1/1
  Switch/1 -> Switch1/3
  Constant3/1 -> Multiport Switch/5, Switch/1
  Constant2/1 -> Multiport Switch/4, Switch/3
  stvHysEngBrkReq/1 -> Switch2/2
  Switch2/1 -> CrCtl_stGearRng_mp/1  "CrCtl_stGearRng_mp"
  Switch1/1 -> Multiport Switch/2, Switch2/3
  Constant5/1 -> Multiport Switch/1
  Multiport Switch/1 -> Switch2/1
